simulink model "lqi"  (R2014b)
settings: Solver=ode4  StartTime=0.0  StopTime=Toss  FixedStep=Ts  RelTol=1e-3
values from neighbouring files (symbols this model uses):
  A = A23    [LQI_LinearizedDynamic_AP2.m]    (also in LQI_LinearizedDynamic_AP2_inputRate.m = [A,B;zeros(nu,nu+nx)]; main.m = sensX*A)
  B = B23    [LQI_LinearizedDynamic_AP2.m]    (also in LQI_LinearizedDynamic_AP2_inputRate.m = [zeros(nx,nu);eye(nu)]; main.m = sensX*B + sensU)
  C = eye(9)    [LQI_LinearizedDynamic_AP2.m]    (also in LQI_LinearizedDynamic_AP2_inputRate.m = eye(nx+nu))
  K_fb = K_aug(:,1:nx)    [LQI_LinearizedDynamic_AP2.m]    (also in LQI_LinearizedDynamic_AP2_inputRate.m)
  K_ff = K_aug(:,nx+1:end)    [LQI_LinearizedDynamic_AP2.m]    (also in LQI_LinearizedDynamic_AP2_inputRate.m)
  nu = length(u0)    [main.m]
  nx = length(x0)    [main.m]
settings Model: Creator=pier  LastModifiedBy=Gianni

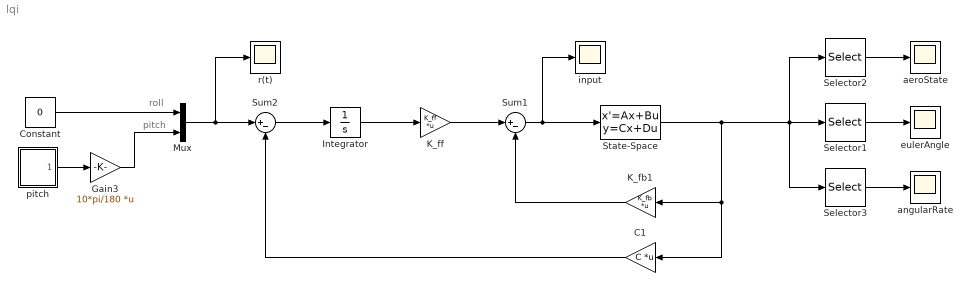
== system lqi ==
  note: pitch
  note: roll
  C1 : Gain  Gain=C  Multiplication=Matrix(K*u)
  Constant : Constant  Value=0
  Gain3 : Gain  Gain=10*pi/180  Multiplication=Matrix(K*u)
  Integrator : Integrator
  K_fb1 : Gain  Gain=K_fb  Multiplication=Matrix(K*u)
  K_ff : Gain  Gain=K_ff  Multiplication=Matrix(K*u)
  Mux : Mux  Inputs=2
  Selector1 : Selector  InputPortWidth=9  Indices=[4:6]
  Selector2 : Selector  InputPortWidth=9  Indices=[1:3]
  Selector3 : Selector  InputPortWidth=9  Indices=[7:9]
  State-Space : StateSpace  A=A  B=B  C=eye(nx)  D=zeros(nx,nu)  X0=0
  Sum1 : Sum  Inputs=|+-
  Sum2 : Sum  Inputs=|+-
  aeroState : Scope
      settings: TimeRange=100  SaveName=sim_aeroState
  angularRate : Scope
      settings: SaveName=sim_angularRate
  eulerAngle : Scope
      settings: TimeRange=10  YMin=-0.025  YMax=0.275  SaveName=sim_eulerAngles
  input : Scope
      settings: TimeRange=100  SaveName=sim_Inputs
  pitch : Subsystem
  r(t) : Scope
      settings: TimeRange=100  SaveName=sim_reference
  wires:
  pitch/1(Out1) -> Gain3/1
  Mux/1 -> Sum2/1, r(t)/1
  Selector1/1 -> eulerAngle/1
  Selector3/1 -> angularRate/1
  Selector2/1 -> aeroState/1
  Sum1/1 -> State-Space/1, input/1
  K_fb1/1 -> Sum1/2
  C1/1 -> Sum2/2
  Sum2/1 -> Integrator/1
  Integrator/1 -> K_ff/1
  K_ff/1 -> Sum1/1
  State-Space/1 -> Selector3/1, Selector1/1, Selector2/1, K_fb1/1, C1/1
  Constant/1 -> Mux/1
  Gain3/1 -> Mux/2

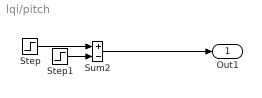
== system lqi/pitch ==
  Step : Step  Time=2.5  SampleTime=0
  Step1 : Step  Time=12.5  SampleTime=0
  Sum2 : Sum  Inputs=+-
  Out1 : Outport
  wires:
  Sum2/1 -> Out1/1
  Step/1 -> Sum2/1
  Step1/1 -> Sum2/2
